simulink model "fahrenheitConverter_StevenJohnson"  (R2025b)
settings: Solver=VariableStepAuto  StartTime=0.0  StopTime=10.0  RelTol=1e-3
libraries: aerolibconvert2 x3

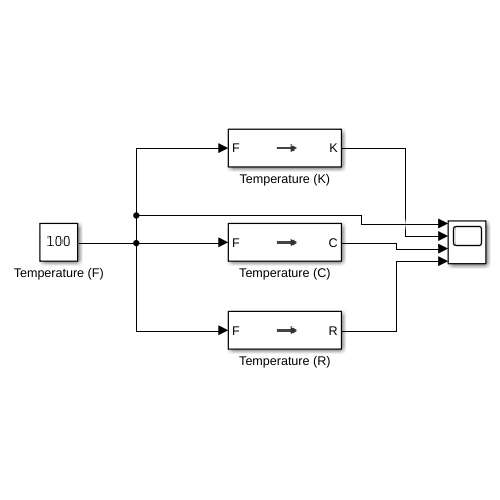
[thumbnail: Simulink's stored preview of the top-level diagram]
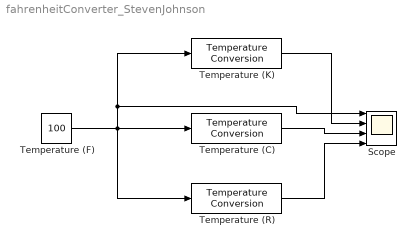
== system fahrenheitConverter_StevenJohnson ==
  Scope : Scope  NumInputPorts=4
      settings: ActiveDisplayYMinimum=-74.208930798762481  ActiveDisplayYMaximum=680.9854238887383  YLabel=Temperature (R,F,K,C)
  Temperature (C) : aerolibconvert2/Temperature Conversion  IU=F  OU=C
  Temperature (F) : Constant  Value=100  SampleTime=0
  Temperature (K) : aerolibconvert2/Temperature Conversion  IU=F  OU=K
  Temperature (R) : aerolibconvert2/Temperature Conversion  IU=F  OU=R
  wires:
  Temperature (R)/1 -> Scope/4
  Temperature (C)/1 -> Scope/3
  Temperature (K)/1 -> Scope/2
  Temperature (F)/1 -> Temperature (R)/1, Temperature (C)/1, Temperature (K)/1, Scope/1
